simulink model "Full_Model"  (R2022b)
settings: Solver=ode23t  StartTime=0.0  StopTime=sim_params.Tstop  FixedStep=1e-4  RelTol=1e-2
undefined symbols (not defined in the file or in its folder): LP_DEN, LP_GAIN, LP_NUM, motor, sim_params
libraries: simulink x2, dspsigops x1
settings Model: Creator=gotta  LastModifiedBy=gotta
settings SolverCC: ZeroCrossAlgorithm=Adaptive
settings DataIOCC: SaveFormat=Array  SignalLogging=off  SaveTime=off  ReturnWorkspaceOutputs=off
settings DebuggingCC: IgnoredZcDiagnostic=none

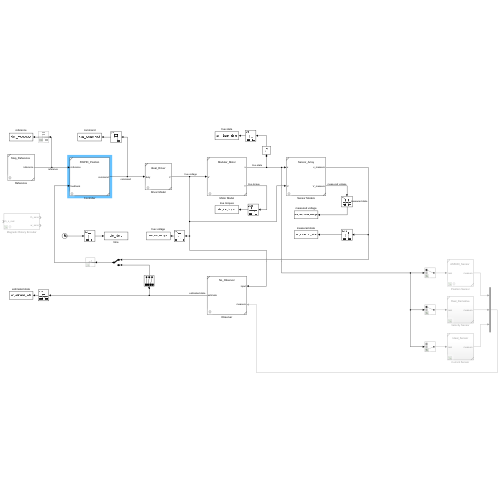
[thumbnail: Simulink's stored preview of the top-level diagram]
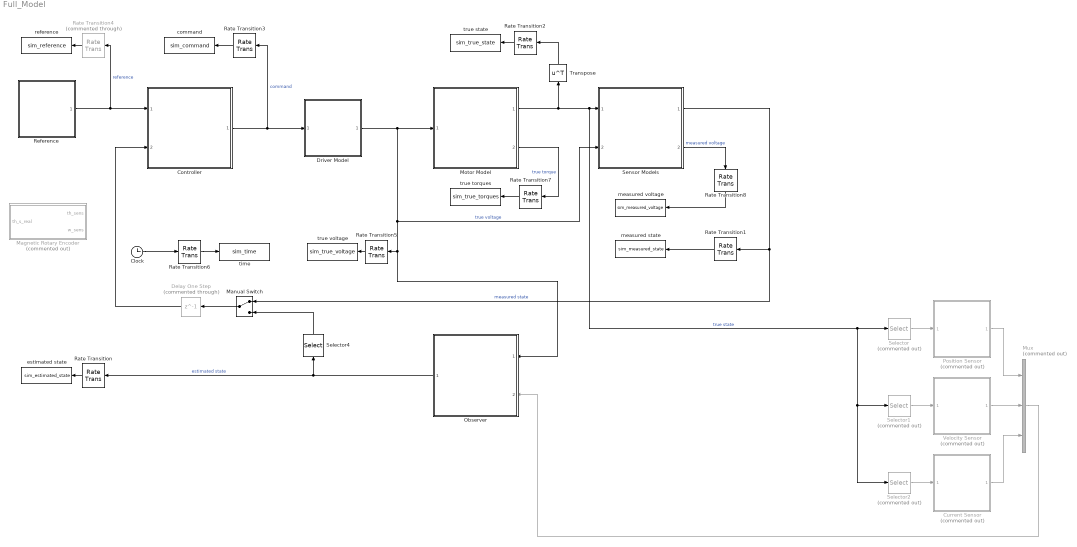
== system Full_Model ==
  Clock : Clock
  Controller : Subsystem  ReferencedSubsystem=SWPID_Position  Kp=10  Ki=0.9  Kd=0.1
  Current Sensor : Subsystem  Commented=on  ReferencedSubsystem=Ideal_Sensor
  Delay One Step : Delay  Commented=through  DelayLength=1  SampleTime=1e-3
  Driver Model : Subsystem  ReferencedSubsystem=Ideal_Driver  driver_model=DRV8830
  Magnetic Rotary Encoder : Subsystem  Commented=on  mask{Vq=motor.Vcc / 2, Va=1.5}
      mask prompts: Vq "Voltage Bias:"; Va "Voltage Amplitude:"
  Manual Switch : ManualSwitch
  Motor Model : Subsystem  ReferencedSubsystem=Modular_Motor  motor_model=motor  initial_conditions=[0;0;0;0]  flux_weakening=on  coulomb_friction=on  stribeck_friction=on
  Mux : Mux  Commented=on  Inputs=3
  Observer : Subsystem  ReferencedSubsystem=No_Observer
  Position Sensor : Subsystem  Commented=on  ReferencedSubsystem=AS5600_Sensor  sensor_model=AS5600  wrapping=off  offset=0
  Rate Transition{,1..3,5..8} (8 alike) : RateTransition  OutPortSampleTime=sim_params.Tsample
  Rate Transition4 : RateTransition  Commented=through  OutPortSampleTime=sim_params.Tsample
  Reference : Subsystem  ReferencedSubsystem=Step_Reference  After=3.1416*10  Time=2
  Selector : Selector  Commented=on  InputPortWidth=3  IndexOptions=Index vector (dialog)  Indices=1  OutputSizes=1
  Selector1 : Selector  Commented=on  InputPortWidth=3  IndexOptions=Index vector (dialog)  Indices=1  OutputSizes=1
  Selector2 : Selector  Commented=on  InputPortWidth=3  IndexOptions=Index vector (dialog)  Indices=3  OutputSizes=1
  Selector4 : Selector  InputPortWidth=4  IndexOptions=Index vector (dialog)  Indices=[1:3]  OutputSizes=1
  Sensor Models : Subsystem  ReferencedSubsystem=Sensor_Array  input1=1  input2=1  input3=3  input4=4
  Transpose : Math  Operator=transpose
  Velocity Sensor : Subsystem  Commented=on  ReferencedSubsystem=Real_Derivative
  command : ToWorkspace  VariableName=sim_command  SampleTime=sim_params.Tsample
      settings: Save2DSignal=2-D array (concatenate along first dimension)
  estimated state : ToWorkspace  VariableName=sim_estimated_state  SampleTime=sim_params.Tsample
      settings: Save2DSignal=2-D array (concatenate along first dimension)
  measured state : ToWorkspace  VariableName=sim_measured_state  SampleTime=sim_params.Tsample
      settings: Save2DSignal=2-D array (concatenate along first dimension)
  measured voltage : ToWorkspace  VariableName=sim_measured_voltage  SampleTime=sim_params.Tsample
      settings: Save2DSignal=2-D array (concatenate along first dimension)
  reference : ToWorkspace  VariableName=sim_reference  SampleTime=sim_params.Tsample
      settings: Save2DSignal=2-D array (concatenate along first dimension)
  time : ToWorkspace  VariableName=sim_time  SampleTime=sim_params.Tsample
      settings: Save2DSignal=2-D array (concatenate along first dimension)
  true state : ToWorkspace  VariableName=sim_true_state  SampleTime=sim_params.Tsample
      settings: Save2DSignal=2-D array (concatenate along first dimension)
  true torques : ToWorkspace  VariableName=sim_true_torques  SampleTime=sim_params.Tsample
      settings: Save2DSignal=2-D array (concatenate along first dimension)
  true voltage : ToWorkspace  VariableName=sim_true_voltage  SampleTime=sim_params.Tsample
      settings: Save2DSignal=2-D array (concatenate along first dimension)
  wires:
  Motor Model/2 -> Rate Transition7/1  "true torque"
  Motor Model/1 -> Selector2/1, Selector1/1, Selector/1, Sensor Models/1, Transpose/1  "true state"
  Sensor Models/1 -> Manual Switch/1, Rate Transition1/1  "measured state"
  Driver Model/1 -> Observer/1, Rate Transition5/1, Sensor Models/2, Motor Model/1  "true voltage"
  Controller/1 -> Rate Transition3/1, Driver Model/1  "command"
  Reference/1 -> Rate Transition4/1, Controller/1  "reference"
  Observer/1 -> Rate Transition/1, Selector4/1  "estimated state"
  Clock/1 -> Rate Transition6/1
  Transpose/1 -> Rate Transition2/1
  Rate Transition/1 -> estimated state/1
  Rate Transition1/1 -> measured state/1
  Rate Transition2/1 -> true state/1
  Rate Transition3/1 -> command/1
  Rate Transition4/1 -> reference/1
  Rate Transition5/1 -> true voltage/1
  Rate Transition6/1 -> time/1
  Rate Transition7/1 -> true torques/1
  Rate Transition8/1 -> measured voltage/1
  Sensor Models/2 -> Rate Transition8/1  "measured voltage"
  Manual Switch/1 -> Delay One Step/1
  Selector4/1 -> Manual Switch/2
  Delay One Step/1 -> Controller/2
  Selector/1 -> Position Sensor/1
  Selector1/1 -> Velocity Sensor/1
  Selector2/1 -> Current Sensor/1
  Position Sensor/1 -> Mux/1
  Velocity Sensor/1 -> Mux/2
  Current Sensor/1 -> Mux/3
  Mux/1 -> Observer/2

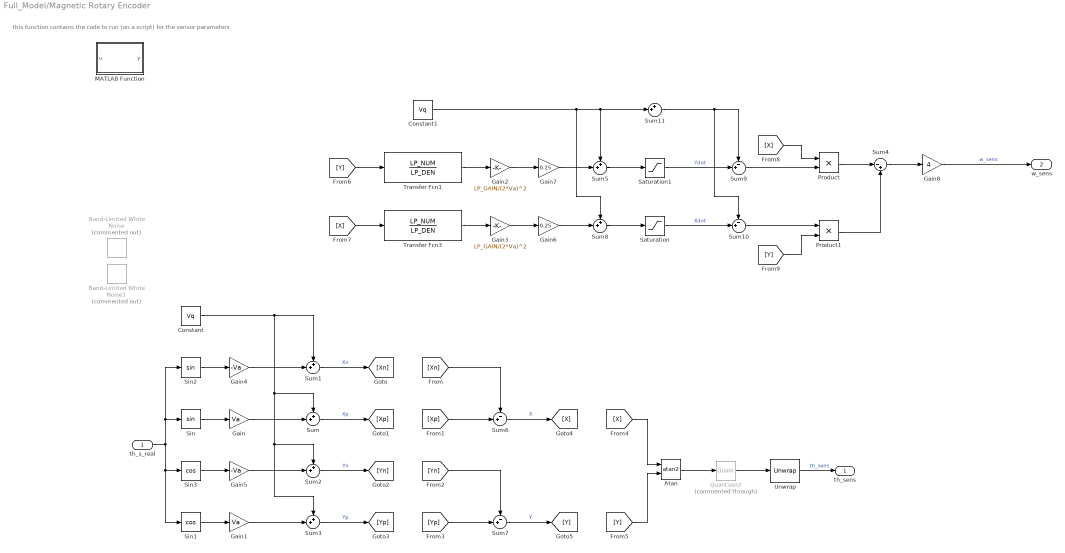
== system Full_Model/Magnetic Rotary Encoder ==
  note: this function contains the code to run (on a script) for the sensor parameters
  th_s_real : Inport
  Atan : Trigonometry  Operator=atan2
  Band-Limited White Noise : simulink/Sources/Band-Limited White Noise  Commented=on  Cov=noise_pwr  Ts=1e-3  seed=[2341]
  Band-Limited White Noise1 : simulink/Sources/Band-Limited White Noise  Commented=on  Cov=noise_pwr  Ts=1e-3  seed=[23541]
  Constant : Constant  Value=Vq
  Constant1 : Constant  Value=Vq
  Gain : Gain  Gain=Va
  Gain1 : Gain  Gain=Va
  Gain2 : Gain  Gain=LP_GAIN/(2*Va)^2
  Gain3 : Gain  Gain=LP_GAIN/(2*Va)^2
  Gain4 : Gain  Gain=-Va
  Gain5 : Gain  Gain=-Va
  Gain6 : Gain  Gain=0.25
  Gain7 : Gain  Gain=0.25
  Gain8 : Gain  Gain=4
  MATLAB Function : MATLAB Function  TreatAsAtomicUnit=on
  Product : Product
  Product1 : Product
  Quantizer2 : Quantizer  Commented=through  QuantizationInterval=AS5600.q_step
  Saturation : Saturate  UpperLimit=4.5  LowerLimit=0.5
  Saturation1 : Saturate  UpperLimit=4.5  LowerLimit=0.5
  Sin : Trigonometry
  Sin1 : Trigonometry  Operator=cos
  Sin2 : Trigonometry
  Sin3 : Trigonometry  Operator=cos
  Sum{,1..3,5,8,11} (7 alike) : Sum  Inputs=++|
  Sum{6..7,9..10} (4 alike) : Sum  Inputs=-+|
  Sum4 : Sum  Inputs=|-+
  Transfer Fcn1 : TransferFcn  Numerator=LP_NUM  Denominator=LP_DEN
  Transfer Fcn3 : TransferFcn  Numerator=LP_NUM  Denominator=LP_DEN
  Unwrap : dspsigops/Unwrap  tol=pi  InputProcessing=Columns as channels (frame based)  running=off
  th_sens : Outport
  w_sens : Outport  Port=2
  wires:
  Sin1/1 -> Gain1/1
  th_s_real/1 -> Sin2/1, Sin/1, Sin1/1, Sin3/1
  Sin/1 -> Gain/1
  Atan/1 -> Quantizer2/1
  Gain/1 -> Sum/2
  Sum4/1 -> Gain8/1
  Gain3/1 -> Gain6/1
  Product1/1 -> Sum4/2
  Product/1 -> Sum4/1
  Transfer Fcn1/1 -> Gain2/1
  Transfer Fcn3/1 -> Gain3/1
  Gain2/1 -> Gain7/1
  Quantizer2/1 -> Unwrap/1
  Sin2/1 -> Gain4/1
  Gain4/1 -> Sum1/2
  Constant/1 -> Sum2/1, Sum3/1, Sum/1, Sum1/1
  Sin3/1 -> Gain5/1
  Gain5/1 -> Sum2/2
  Gain1/1 -> Sum3/2
  Sum1/1 -> [Xn]  "Xn"
  Sum/1 -> [Xp]  "Xp"
  Sum2/1 -> [Yn]  "Yn"
  Sum3/1 -> [Yp]  "Yp"
  [Xp] -> Sum6/2
  [Xn] -> Sum6/1
  [Yn] -> Sum7/1
  [Yp] -> Sum7/2
  Sum6/1 -> [X]  "X"
  Sum7/1 -> [Y]  "Y"
  [Y] -> Transfer Fcn1/1
  [X] -> Transfer Fcn3/1
  [X] -> Atan/1
  [Y] -> Atan/2
  Unwrap/1 -> th_sens/1  "th_sens"
  Saturation/1 -> Sum10/2  "Xdot"
  Saturation1/1 -> Sum9/2  "Ydot"
  Constant1/1 -> Sum8/1, Sum11/2, Sum5/1
  Sum5/1 -> Saturation1/1
  Sum8/1 -> Saturation/1
  [X] -> Product/1
  Sum9/1 -> Product/2
  Sum10/1 -> Product1/1
  [Y] -> Product1/2
  Gain6/1 -> Sum8/2
  Gain7/1 -> Sum5/2
  Gain8/1 -> w_sens/1  "w_sens"
  Sum11/1 -> Sum10/1, Sum9/1

== matlab function Full_Model/Magnetic Rotary Encoder/MATLAB Function ==
  data: u input; y output
function y = fcn(u)

% Low Speed Tachometer Parameters
s = tf('s');
wn = 50*2*pi;           % cutoff frequency [Hz]
csi = 1/sqrt(2);        % damping coefficient

lowpass = s / (s^2 + 2*csi*wn*s + wn^2);
[LP_NUM, LP_DEN] = tfdata(lowpass);
LP_NUM = cell2mat(LP_NUM);
LP_DEN = cell2mat(LP_DEN);

[LP_MAG, LP_PHASE] = bode(lowpass, 1);
LP_GAIN = 1/LP_MAG;

noise_pwr = 1e-7;

% Discrete Lowpass Filter Parameters
fc = 50; % cutoff frequency [Hz]
Fs = 1e3; % sampling frequency [Hz]

wc = 2*pi*fc / Fs;
a = 1 - exp(-wc);

numd = [a 0];
dend = [1 a-1];


y = u;
